simulink model "simProcObsSquare"  (Simulink 9.3)
settings: Solver=FixedStepAuto  StartTime=0.0  StopTime=2  FixedStep=0.002  RelTol=1e-3
values from neighbouring files (symbols this model uses):
  A = [-4 -0.03; 0.75 -10]    [MDLsisotool.m]    (also in arq1_23_04_19.m; dadosSS.mat = [-31.7879344999  -235.758689997; 1  0]; dadosSS3.mat = [-672.744698351  -20610.4503166  -151111.126991; 1  0  0; 0 )
  B = [2; 0]    [MDLsisotool.m]    (also in arq1_23_04_19.m; dadosSS.mat = [1 0]; dadosSS3.mat = [1 0 0])
  C = [0 1]    [MDLsisotool.m]    (also in arq1_23_04_19.m; dadosSS.mat = [0 -5669.87734101]; dadosSS3.mat = [0 0 3634146.23193])
  D = 0    [MDLsisotool.m]    (also in arq1_23_04_19.m; dadosSS.mat; dadosSS3.mat)
  Ki = Kext(3)    [MDLsspace.m]    (also in dadosSS.mat = 0.0370378382758; dadosSS3.mat = -0.00217932892475; ssGera.m = Kext(4))
  Kproc = [Kext(1), Kext(2)]    [MDLsspace.m]    (also in dadosSS.mat = [-13.7879344999 -128.758689997]; dadosSS3.mat = [-634.744698351 -20071.4503166 -147729.126991]; ssGera.m = [Kext(1), Kext(2), Kext(3)])
  L = (acker(A', C', polosObs))'    [MDLsspace.m]    (also in dadosSS.mat = [0.0267900926393 -0.00885593505471]; dadosSS3.mat = [-62.4863664427 0.0974835238697 -0.000151272035649]; ssGera.m)
settings Model: Creator=Cadu  LastModifiedBy=Cadu
settings DataIOCC: SaveFormat=Dataset  SignalLoggingSaveFormat=Dataset  ReturnWorkspaceOutputs=on
settings OptimizationCC: LifeSpan=auto
settings DebuggingCC: UnderspecifiedInitializationDetection=Simplified  MergeDetectMultiDrivingBlocksExec=error  FcnCallInpInsideContextMsg=error  SFUnexpectedBacktrackingDiag=error  SFNoUnconditionalDefaultTransitionDiag=error  SFExecutionAtInitializationDiag=warning  ArithmeticOperatorsInVariantConditions=error
settings HardwareCC: ProdBitPerPointer=64  ProdBitPerSizeT=64  ProdBitPerPtrDiffT=64  ProdLargestAtomicFloat=Float  ProdIntDivRoundTo=Zero  ProdEndianess=LittleEndian  ProdWordSize=64  ProdHWDeviceType=Intel->x86-64 (Windows64)
settings ModelReferenceCC: PropagateSignalLabelsOutOfModel=on
settings SFSimCC: SimUseLocalCustomCode=on
settings RTWCC: RTWUseLocalCustomCode=on
settings CodeAppCC: StateflowObjectComments=off
settings GRTTargetCC: TargetLangStandard=C99 (ISO)  CombineOutputUpdateFcns=on  GRTInterface=off
settings ConfigComp: CovMetricSettings=dwe  CovHtmlReporting=off  CovSaveCumulativeToWorkspaceVar=off  CovSaveSingleToWorkspaceVar=off  CovExternalEMLEnable=on

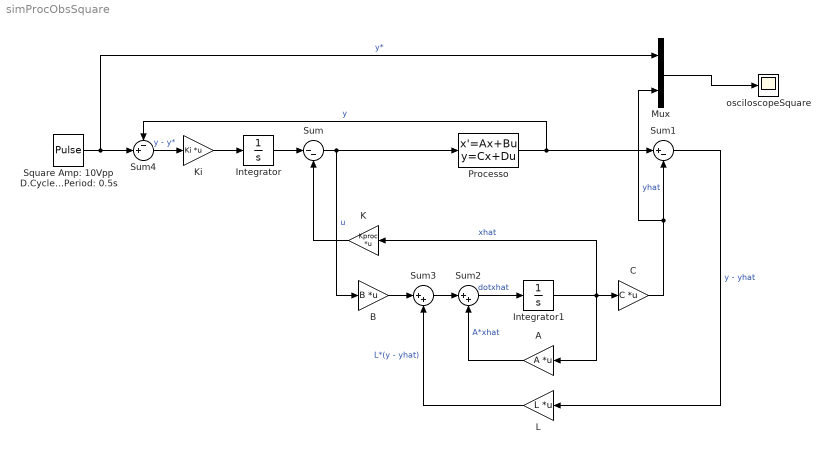
== system simProcObsSquare ==
  " A" : Gain  Gain=A  Multiplication=Matrix(K*u)
  " K" : Gain  Gain=Kproc  Multiplication=Matrix(K*u)
  "B " : Gain  Gain=B  Multiplication=Matrix(K*u)
  C : Gain  Gain=C  Multiplication=Matrix(K*u)
  Integrator : Integrator
  Integrator1 : Integrator
  Ki : Gain  Gain=Ki  Multiplication=Matrix(K*u)
  "L " : Gain  Gain=L  Multiplication=Matrix(K*u)
  Mux : Mux  Inputs=2
  "Processo " : StateSpace  A=A  B=B  C=C  D=D  InitialCondition=0
  Square Amp: 10Vpp D.Cycle: 50% Period: 0.5s : DiscretePulseGenerator  PulseType=Time based  Amplitude=5  Period=0.5  PulseWidth=50
  Sum : Sum  Inputs=|--
  Sum1 : Sum  Inputs=|+-
  Sum2 : Sum  Inputs=|++
  Sum3 : Sum  Inputs=|++
  Sum4 : Sum  Inputs=-+|
  osciloscopeSquare : Scope
  wires:
  Sum/1 -> "Processo "/1, "B "/1  "u"
  Integrator/1 -> Sum/1
  "Processo "/1 -> Sum1/1, Sum4/1  "y"
  Sum1/1 -> "L "/1  "y - yhat"
  Integrator1/1 -> " A"/1, C/1, " K"/1  "xhat"
  Sum2/1 -> Integrator1/1  "dotxhat"
  " K"/1 -> Sum/2
  Sum3/1 -> Sum2/1
  "B "/1 -> Sum3/1
  C/1 -> Mux/2, Sum1/2  "yhat"
  " A"/1 -> Sum2/2  "A*xhat"
  "L "/1 -> Sum3/2  "L*(y - yhat)"
  Ki/1 -> Integrator/1
  Mux/1 -> osciloscopeSquare/1
  Square Amp: 10Vpp D.Cycle: 50% Period: 0.5s/1 -> Sum4/2, Mux/1  "y*"
  Sum4/1 -> Ki/1  "y - y*"
